simulink model "turbine_decoupled"  (R2025b)
settings: Solver=FixedStepAuto  StartTime=0.0  StopTime=399  FixedStep=Ts_inner  RelTol=1e-3
InitFcn:
  | turbine_model_constants;
values from neighbouring files (symbols this model uses):
  A = Simulink.Parameter(R.Value^2*pi)    [turbine_model_constants.m]
  beta_opt_vector = Simulink.Parameter(beta_array)    [turbine_model_constants.m]
  beta_vector = Simulink.Parameter(tables{4})    [turbine_model_constants.m]
  c_beta_dot = Simulink.Parameter(0.5)    [turbine_model_constants.m]
  c_gamma_dot = Simulink.Parameter(0.5/180*pi)    [turbine_model_constants.m]
  cp_max = Simulink.Parameter(max(cp_table.Value(:))*0.99)    [turbine_model_constants.m]
  cp_opt_keys = Simulink.Parameter(cell2mat(cp_vector))    [turbine_model_constants.m]
  cp_table = Simulink.Parameter(tables{1})    [turbine_model_constants.m]
  ct_table = Simulink.Parameter(tables{2})    [turbine_model_constants.m]
  JT = Simulink.Parameter(2.052*10^8*3)    [turbine_model_constants.m]
  lambda_opt_vector = Simulink.Parameter(lambda_array)    [turbine_model_constants.m]
  lambda_vector = Simulink.Parameter(tables{5})    [turbine_model_constants.m]
  mu = Simulink.Parameter(0.95)    [turbine_model_constants.m]
  R = Simulink.Parameter(142)    [turbine_model_constants.m]
  rho = Simulink.Parameter(1.225)    [turbine_model_constants.m]
  Ts = 1    [turbine_model_constants.m]
  Ts_inner = Simulink.Parameter(0.1)    [turbine_model_constants.m]
undefined symbols (not defined in the file or in its folder): DiscIntNeverNeededParam, f
libraries: instrumentlib x2, slpidlib x1
settings Model: Creator=kohlh  LastModifiedBy=kohlh

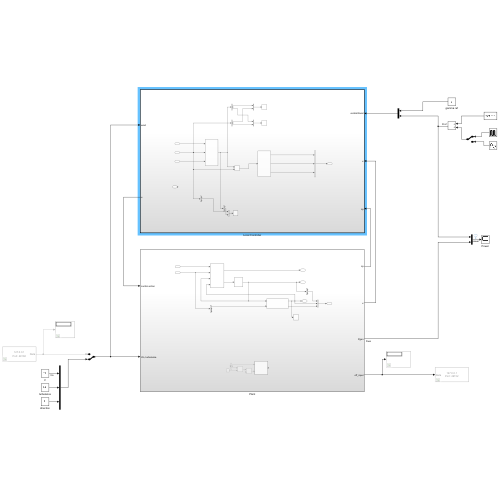
[thumbnail: Simulink's stored preview of the top-level diagram]
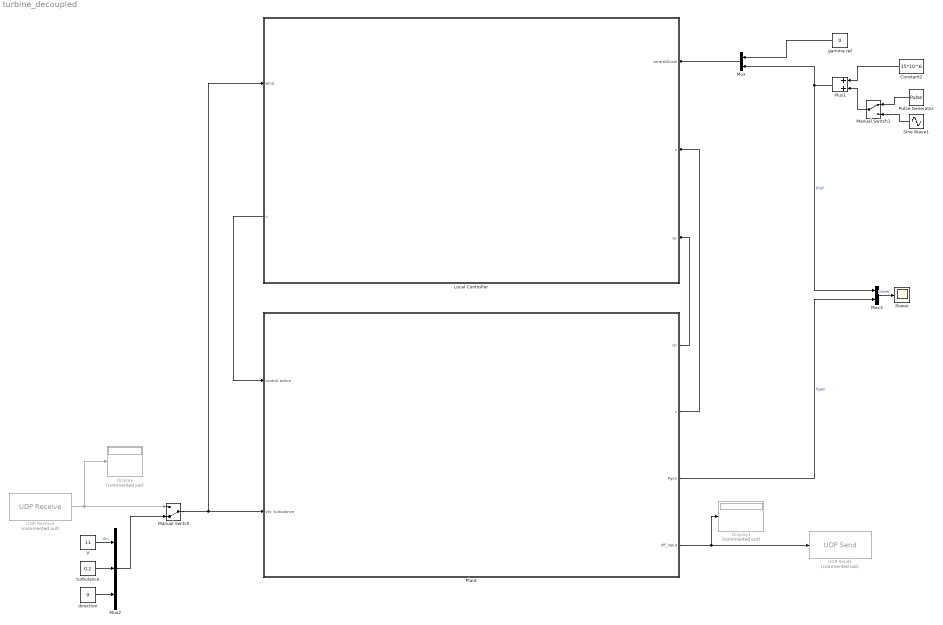
== system turbine_decoupled ==
  Constant2 : Constant  Value=15*10^6
  Display : Display  Commented=on
  Display1 : Display  Commented=on
  Local Controller : Subsystem  TreatAsAtomicUnit=on
      settings: PortSchema="{\"entries\":[{\"content\":{\"sides\":[{\"content\":{\"connectorIds\":[\"In1\",\"In2\",\"In3\"]},\"type\":\"ConnectorPlacement.EquallySpacedRectSide\",\"uuid\":\"1274bf49-ceae-40b5-8168-864c275c8277\"},{\"content\":{\"connectorIds\":[\"In4\",\"Out1\"],\"side\":\"RIGHT\"},\"type\":\"ConnectorPlacement.EquallySpacedRectSide\",\"uuid\":\"983d855e-2fb7-4029-8a1e-74d0395d6e6b\"},{\"content\":{\"side\":\"TOP\"},\"type\":\"ConnectorPlacement.EquallySpacedRectSide\",\"uuid\":\"78e40a3c-46aa-4158-bc61-97e5b88f823b\"},{\"content\":{\"side\":\"BOTTOM\"},\"type\":\"ConnectorPlacement.EquallySpacedRectSide\",\"uuid\":\"db79cd87-5583-4254-9385-067380eca232\"}]},\"type\":\"ConnectorPlacement.EquallySpacedConnector\",\"uuid\":\"902a270f-1fdc-458f-b9eb-4015978e6616\"}],\"packageUris\":[\"http://schema.mathworks.com/mf0/Connector/R2020b\"],\"version\":\"1.0\"}"
  Manual Switch : ManualSwitch  CurrentSetting=0
  Manual Switch1 : ManualSwitch
  Mux : Mux  Inputs=2
  Mux2 : Mux  Inputs=3
  Mux3 : Mux  Inputs=2
  Plant : Subsystem
  Plus1 : Sum
  Power : Scope
      settings: ActiveDisplayYMinimum=-8.3745470708276331E+6  ActiveDisplayYMaximum=3.1326975350164406E+7  DataLoggingVariableName=ScopeData4
  Pulse Generator : DiscretePulseGenerator  PulseType=Time based  Amplitude=5*10^6  Period=400  PulseWidth=50
  Sine Wave1 : Sin  Amplitude=5*10^6  Frequency=3.24/1000  SampleTime=0
  UDP Receive : instrumentlib/UDP Receive  Commented=on  LocalAddress=127.0.0.1  LocalPort=49160  EnablePortSharing=off  Host=127.0.0.1  Port=49152  GetLatestData=off  DataSize=3  DataType=double  ASCIIFormatting=%f,  Terminator=LF  CustomTerminator=10  ByteOrder=big-endian  EnableBlockingMode=on  Timeout=10  SampleTime=Ts  SimulateUsing=Interpreted execution
  UDP Send1 : instrumentlib/UDP Send  Commented=on  Host=127.0.0.1  Port=49152  LocalAddress=0.0.0.0  LocalPort=-1  EnablePortSharing=off  OutputDatagramPacketSize=512  ByteOrder=big-endian  EnableBlockingMode=on  SimulateUsing=Interpreted execution
  V : Constant  Value=11
  direction : Constant  Value=0
  gamma ref : Constant  Value=0
  turbulance : Constant  Value=0.2
  wires:
  Plant/2(x) -> Local Controller/2(x)
  Local Controller/1(u) -> Plant/1(control action)
  Plant/3(Pgen) -> Mux3/2  "Pgen"
  Manual Switch/1 -> Local Controller/4(wind), Plant/2("Vin, turbulance")
  Manual Switch1/1 -> Plus1/2
  Sine Wave1/1 -> Manual Switch1/2
  Constant2/1 -> Plus1/1
  V/1 -> Mux2/1  "Vin"
  turbulance/1 -> Mux2/2
  Mux3/1 -> Power/1  "power"
  Plant/1(cp) -> Local Controller/3(cp)
  Pulse Generator/1 -> Manual Switch1/1
  direction/1 -> Mux2/3
  Mux2/1 -> Manual Switch/2
  Plus1/1 -> Mux/2, Mux3/1  "Pref"
  gamma ref/1 -> Mux/1
  Mux/1 -> Local Controller/1(central2local)
  Plant/4(off_input) -> Display1/1, UDP Send1/1
  UDP Receive/1 -> Manual Switch/1, Display/1

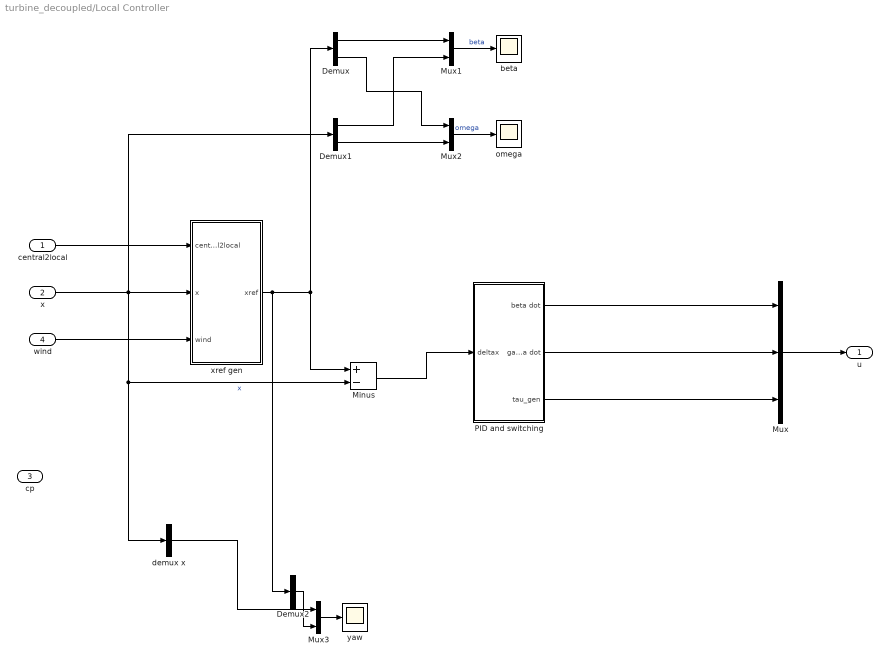
== system turbine_decoupled/Local Controller ==
  central2local : Inport
  x : Inport  Port=2
  cp : Inport  Port=3
  wind : Inport  Port=4
  Demux : Demux  Outputs=3
  Demux1 : Demux  Outputs=3
  Demux2 : Demux  Outputs=3
  Minus : Sum  Inputs=+-
  Mux : Mux  Inputs=3
  Mux1 : Mux  Inputs=2
  Mux2 : Mux  Inputs=2
  Mux3 : Mux  Inputs=2
  PID and switching : Subsystem
  beta : Scope
      settings: ActiveDisplayYMinimum=-0.675  ActiveDisplayYMaximum=6.0750000000000011
  demux x : Demux  Outputs=3
  omega : Scope
      settings: ActiveDisplayYMinimum=-0.34183960096413279  ActiveDisplayYMaximum=3.0765564086771957
  xref gen : MATLAB Function  TreatAsAtomicUnit=on
  yaw : Scope
      settings: ActiveDisplayYMinimum=-5.7595100216969257  ActiveDisplayYMaximum=9.1647979110356328  DataLoggingVariableName=ScopeData3
  u : Outport
  wires:
  central2local/1 -> xref gen/1(central2local)
  xref gen/1(xref) -> Demux2/1, Minus/1, Demux/1
  Mux/1 -> u/1
  PID and switching/1(beta dot) -> Mux/1
  PID and switching/2(gamma dot) -> Mux/2
  x/1 -> demux x/1, Minus/2, Demux1/1, xref gen/2(x)  "x"
  wind/1 -> xref gen/3(wind)
  Mux1/1 -> beta/1  "beta"
  Mux2/1 -> omega/1  "omega"
  Demux/1 -> Mux1/1
  Demux1/3 -> Mux2/2
  Demux1/1 -> Mux1/2
  Demux/3 -> Mux2/1
  demux x/2 -> Mux3/1
  Mux3/1 -> yaw/1
  Demux2/2 -> Mux3/2
  Minus/1 -> PID and switching/1(deltax)
  PID and switching/3(tau_gen) -> Mux/3

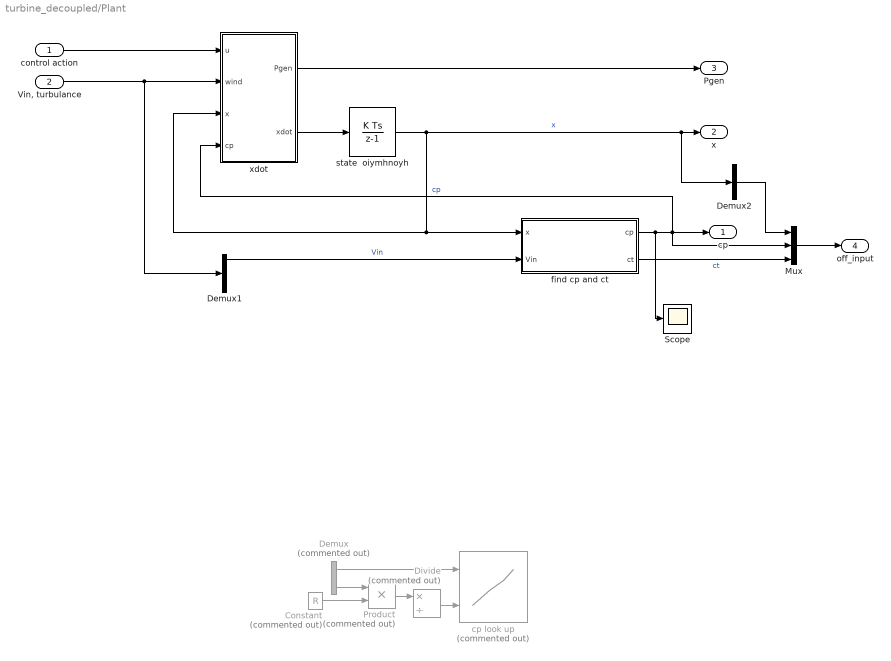
== system turbine_decoupled/Plant ==
  control action : Inport
  "Vin, turbulance" : Inport  Port=2
  Constant : Constant  Commented=on  Value=R
  Demux : Demux  Commented=on  Outputs=3
  Demux1 : Demux  Outputs=3
  Demux2 : Demux  Outputs=3
  Divide : Product  Commented=on  Inputs=*/
  Mux : Mux  Inputs=3
  Product : Product  Commented=on
  Scope : Scope
      settings: ActiveDisplayYMinimum=-0.044951731714988244  ActiveDisplayYMaximum=0.53080020994082311  DataLoggingVariableName=ScopeData2
  cp look up : Lookup_n-D  Commented=on  BreakpointsForDimension1="[2.0    2.632    3.263    3.895    4.526    5.158    5.789    6.421    7.053    7.684    8.316    8.947    9.579    10.21    10.84    11.47    12.11    12.74    13.37    14.0]"  BreakpointsForDimension2="[-5.0   -2.368   0.2632   2.895   5.526   8.158   10.79   13.42   16.05   18.68   21.32   23.95   26.58   29.21   31.84   34.47   37.11   39.74   42.37   45.0]"  Table=|  ExtrapMethod=Clip  UseLastTableValue=on  InternalRulePriority=Speed  RndMeth=Simplest
      | [0.004183   0.008552   0.013076   0.017954   0.023246   0.028797   0.034398   0.040294   0.047129   0.053808   0.057993   0.058951   0.056907   0.052360   0.045879   0.038003   0.029036   0.019157   0.008446   -0.002755;   
      | 0.014528   0.023851   0.033841   0.044146   0.054123   0.065155   0.078342   0.088804   0.092608   0.090398   0.083572   0.073569   0.061407   0.047713   0.032764   0.016578   -0.000877   -0.018725   -0.033888   -0.044500   ;
      | 0.035083   0.052168   0.068563   0.085329   0.106367   0.126719   0.134796   0.131887   0.121585   0.106602   0.088719   0.068791   0.047244   0.024090   -0.000932   -0.027634   -0.052318   -0.069329   -0.080611   -0.089918   ;
      | 0.067497   0.092129   0.118436   0.152867   0.179485   0.184226   0.174698   0.156824   0.134064   0.108187   0.079927   0.049652   0.017175   -0.018082   -0.055707   -0.088857   -0.109352   -0.123217   -0.135333   -0.145575   ;
      | 0.109296   0.146828   0.196926   0.234101   0.238344   0.224125   0.199908   0.169919   0.136059   0.099086   0.059484   0.016949   -0.029396   -0.079729   -0.125829   -0.154070   -0.171841   -0.188440   -0.202090   -0.218450   ;
      | 0.163377   0.228953   0.285997   0.296203   0.280800   0.252396   0.216375   0.175204   0.129721   0.080591   0.027761   -0.029928   -0.093612   -0.157541   -0.201469   -0.225214   -0.247672   -0.266413   -0.286681   -0.311430   ;
      | 0.239912   0.324864   0.352474   0.342011   0.313180   0.273733   0.226976   0.174102   0.115954   0.053053   -0.015678   -0.091943   -0.174928   -0.244852   -0.282403   -0.310236   -0.337440   -0.361077   -0.393459   -0.426107   ;
      | 0.333600   0.395237   0.400481   0.377508   0.339368   0.290473   0.232755   0.167308   0.095180   0.016217   -0.071529   -0.170062   -0.270275   -0.338551   -0.374587   -0.411011   -0.442593   -0.477339   -0.524911   -0.565339   ;
      | 0.402440   0.440975   0.435173   0.406148   0.361342   0.303497   0.234290   0.155195   0.067363   -0.030370   -0.140598   -0.264045   -0.376585   -0.440727   -0.482770   -0.527917   -0.566739   -0.618765   -0.682470   -0.732169   ;
      | 0.432644   0.465056   0.459322   0.429497   0.379883   0.313246   0.231892   0.137909   0.032249   -0.087249   -0.223737   -0.372811   -0.492396   -0.554948   -0.608268   -0.662234   -0.713574   -0.787600   -0.867515   -0.929642   ;
      | 0.422710   0.465336   0.473606   0.448041   0.395244   0.319950   0.225727   0.115425   -0.010492   -0.155017   -0.321542   -0.495464   -0.618709   -0.684596   -0.751969   -0.816482   -0.886063   -0.985630   -1.082210   -1.161646   ;
      | 0.396284   0.443496   0.476394   0.461471   0.407453   0.323743   0.215870   0.087597   -0.061232   -0.234314   -0.434191   -0.631316   -0.757268   -0.831922   -0.915179   -0.993282   -1.086290   -1.214677   -1.328998   -1.433710   ;
      | 0.364006   0.418141   0.464679   0.468984   0.416461   0.324694   0.202328   0.054221   -0.120379   -0.325817   -0.561780   -0.780269   -0.909948   -0.998339   -1.099511   -1.194694   -1.316095   -1.476528   -1.610379   -1.752233   ;
      | 0.325277   0.390074   0.445602   0.469191   0.422138   0.322825   0.185054   0.015070   -0.188371   -0.430168   -0.704475   -0.942914   -1.078621   -1.185143   -1.306571   -1.422529   -1.577451   -1.773037   -1.929044   -2.123730   ;
      | 0.279585   0.358093   0.423416   0.460215   0.424264   0.318123   0.163968   -0.030112   -0.265678   -0.547899   -0.862513   -1.120134   -1.265031   -1.393761   -1.537797   -1.678629   -1.872403   -2.106073   -2.288499   -2.553238   ;
      | 0.226506   0.321424   0.398243   0.444906   0.422523   0.310551   0.138956   -0.081606   -0.352786   -0.679510   -1.036172   -1.312951   -1.470710   -1.625580   -1.794579   -1.964822   -2.202969   -2.477562   -2.692792   -3.044259   ;
      | 0.165936   0.279533   0.369843   0.426424   0.416456   0.300051   0.109877   -0.139708   -0.450192   -0.825504   -1.225802   -1.522456   -1.697101   -1.881847   -2.078375   -2.282902   -2.571085   -2.889486   -3.146140   -3.599615   ;
      | 0.099525   0.232060   0.337924   0.405286   0.405362   0.286537   0.076570   -0.204724   -0.558401   -0.986390   -1.431931   -1.749759   -1.945607   -2.163742   -2.390678   -2.634632   -2.978667   -3.343918   -3.652816   -4.221737   ;
      | 0.037721   0.178916   0.302216   0.381569   0.388958   0.269906   0.038866   -0.276967   -0.677907   -1.162688   -1.655209   -1.995993   -2.217511   -2.472435   -2.732975   -3.021755   -3.427648   -3.842988   -4.217100   -4.912785   ;
      | -0.007435   0.121264   0.262494   0.355204   0.368798   0.250044   -0.003414   -0.356756   -0.809181   -1.354921   -1.896339   -2.262341   -2.513981   -2.809119   -3.106746   -3.446005   -3.919962   -4.388970   -4.843093   -5.674879]
      settings: InputPortMap=u0,u1
  find cp and ct : MATLAB Function  TreatAsAtomicUnit=on
  state  oiymhnoyh : DiscreteIntegrator  InitialCondition=[0,0,0]  SampleTime=-1  ICPrevOutput=DiscIntNeverNeededParam  ICPrevScaledInput=DiscIntNeverNeededParam
  xdot : MATLAB Function  TreatAsAtomicUnit=on
  cp : Outport
  x : Outport  Port=2
  Pgen : Outport  Port=3
  off_input : Outport  Port=4
  wires:
  "Vin, turbulance"/1 -> xdot/2(wind), Demux1/1
  xdot/2(xdot) -> state  oiymhnoyh/1
  state  oiymhnoyh/1 -> Demux2/1, x/1, find cp and ct/1(x), xdot/3(x)  "x"
  control action/1 -> xdot/1(u)
  Demux/1 -> cp look up/1
  Demux/3 -> Product/1
  Constant/1 -> Product/2
  Product/1 -> Divide/1
  Divide/1 -> cp look up/2
  xdot/1(Pgen) -> Pgen/1
  Demux1/1 -> find cp and ct/2(Vin)  "Vin"
  find cp and ct/1(cp) -> Scope/1, Mux/2, cp/1, xdot/4(cp)  "cp"
  find cp and ct/2(ct) -> Mux/3  "ct"
  Demux2/2 -> Mux/1
  Mux/1 -> off_input/1

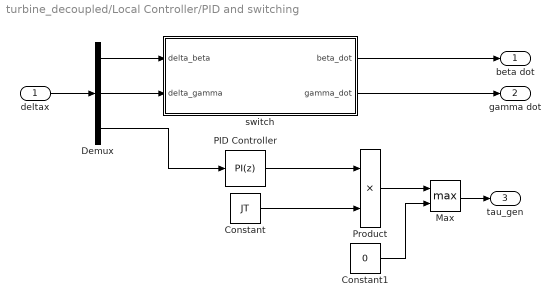
== system turbine_decoupled/Local Controller/PID and switching ==
  deltax : Inport
  Constant : Constant  Value=JT
  Constant1 : Constant  Value=0
  Demux : Demux  Outputs=3
  Max : MinMax  Function=max  Inputs=2
  PID Controller : slpidlib/PID Controller  Controller=PI  Form=Parallel  TimeDomain=Discrete-time  UseExternalTs=off  SampleTime=-1  IntegratorMethod=Forward Euler  FilterMethod=Forward Euler  ControllerParametersSource=internal  P=-0.01  I=-0.001  UseKiTs=off  D=0  UseExternalDerivativeSource=off  N=100  UseFilter=on  TunerSelectOption=Transfer Function Based (PID Tuner App)  InitialConditionSource=internal  InitialConditionForIntegrator=0  InitialConditionForFilter=0  DifferentiatorICPrevScaledInput=0  ExternalReset=none  TrackingMode=off  Kt=1  LimitOutput=off  SatLimitsSource=internal  UpperSaturationLimit=inf  LowerSaturationLimit=-inf  LinearizeAsGain=on  AntiWindupMode=none  Kb=1  LimitIntegrator=off  UpperIntegratorSaturationLimit=inf  LowerIntegratorSaturationLimit=-inf  POutMin=[]  POutMax=[]  IOutMin=[]  IOutMax=[]  DOutMin=[]  DOutMax=[]  NOutMin=[]  NOutMax=[]  SumOutMin=[]  SumOutMax=[]  SaturationOutMin=[]  SaturationOutMax=[]  PParamMin=[]  PParamMax=[]  IParamMin=[]  IParamMax=[]  DParamMin=[]  DParamMax=[]  NParamMin=[]  NParamMax=[]  KbParamMin=[]  KbParamMax=[]  KtParamMin=[]  KtParamMax=[]  KbOutMin=[]  KbOutMax=[]  KtOutMin=[]  KtOutMax=[]  IntegratorOutMin=[]  IntegratorOutMax=[]  FilterOutMin=[]  FilterOutMax=[]  SumI1OutMin=[]  SumI1OutMax=[]  SumI2OutMin=[]  SumI2OutMax=[]  SumI3OutMin=[]  SumI3OutMax=[]  SumI4OutMin=[]  SumI4OutMax=[]  SumDOutMin=[]  SumDOutMax=[]  DifferentiatorOutMin=[]  DifferentiatorOutMax=[]  FilterDiffOutCoefMin=[]  FilterDiffOutCoefMax=[]  ReciprocalOutMin=[]  ReciprocalOutMax=[]  SumDenOutMin=[]  SumDenOutMax=[]  SumNumOutMin=[]  SumNumOutMax=[]  DivideOutMin=[]  DivideOutMax=[]  UdiffTsProdOutMin=[]  UdiffTsProdOutMax=[]  NTsProdOutMin=[]  NTsProdOutMax=[]  UintegralTsProdOutMin=[]  UintegralTsProdOutMax=[]  UngainTsProdOutMin=[]  UngainTsProdOutMax=[]  ClampingZeroOutDataTypeStr=Inherit: Inherit via back propagation  ClampingZeroOutMin=[]  ClampingZeroOutMax=[]  FilterDenConstantOutDataTypeStr=Inherit: Inherit via back propagation  FilterDenConstantOutMin=[]  FilterDenConstantOutMax=[]  PCopyOutDataTypeStr=Inherit: Inherit via back propagation  PCopyOutMin=[]  PCopyOutMax=[]  NCopyOutDataTypeStr=Inherit: Inherit via back propagation  NCopyOutMin=[]  NCopyOutMax=[]  IntegratorContinuousStateAttributes=''  IntegratorStateMustResolveToSignalObject=off  IntegratorRTWStateStorageClass=Auto  FilterContinuousStateAttributes=''  FilterStateMustResolveToSignalObject=off  FilterRTWStateStorageClass=Auto  ParallelPVariant=InternalParameters  IdealPVariant=Disabled  IVariant=InternalParameters  DVariant=Disabled  IntegratorVariant=Discrete  SatVariant=Disabled  AWVariant=Passthrough  PCopyVariant=Disabled  TRVariant=Disabled  FdbkBlocksVariant=Forward  IdealPFdbkVariant=Disabled  SatFdbkVariant=Disabled  DerivativeFilterVariant=Disabled  NVariant=Disabled  NCopyVariant=Disabled_SignalSpec  FilterICVariant=Disabled  IntegratorICVariant=InternalICs  ExternalResetVariant=Disabled  TRSumVariant=Passthrough  SumFdbkVariant=Disabled  SumVariant=Sum_PI  TsampFilterVariant=InternalTs  TsampNgainVariant=Passthrough  TsampIntegralVariant=Disabled_SignalSpec  ExternalSaturationOutDataTypeStr=Inherit: Same as second input  DerivativeSourceVariant=Disabled  PreIntVariant=InternalPreInt
  Product : Product
  switch : MATLAB Function  TreatAsAtomicUnit=on
  beta dot : Outport
  gamma dot : Outport  Port=2
  tau_gen : Outport  Port=3
  wires:
  deltax/1 -> Demux/1
  Demux/1 -> switch/1(delta_beta)
  Demux/2 -> switch/2(delta_gamma)
  switch/2(gamma_dot) -> gamma dot/1
  switch/1(beta_dot) -> beta dot/1
  Demux/3 -> PID Controller/1
  PID Controller/1 -> Product/1
  Constant/1 -> Product/2
  Product/1 -> Max/1
  Constant1/1 -> Max/2
  Max/1 -> tau_gen/1

== matlab function turbine_decoupled/Local Controller/PID and switching/switch ==
  data: beta_dot output; delta_beta input; gamma_dot output; delta_gamma input; c_beta_dot parameter; c_gamma_dot parameter; Ts_inner parameter
function [beta_dot, gamma_dot]= switch_controller(delta_beta, delta_gamma, c_beta_dot, c_gamma_dot, Ts_inner)


if abs(delta_beta) > 0.5*Ts_inner*c_beta_dot
    if delta_beta > 0
        beta_dot = c_beta_dot;
    else
        beta_dot = -c_beta_dot;
    end
else
    beta_dot = 0;
end

if abs(delta_gamma) > 0.5*Ts_inner*c_gamma_dot
    if delta_gamma > 0
        gamma_dot = c_gamma_dot;
    else
        gamma_dot = -c_gamma_dot;
    end
else
    gamma_dot = 0;
end

end

== matlab function turbine_decoupled/Plant/xdot ==
  data: Pgen output; u input; xdot output; wind input; x input; cp input; JT parameter; A parameter; rho parameter; mu parameter
function [Pgen, xdot] = fcn(u, wind, x, cp, JT, A, rho, mu)

Vin = wind(1);
turbulance = 1-wind(2);
wind_direction = wind(3);

beta_dot = u(1);
gamma_dot = u(2);
tau_gen = u(3);

gamma = x(2);
omega = x(3);

%eliminating division by 0
if omega < 0.1 && omega >= 0
    omega = 0.1;
    tau_gen = 0;
    % if there is no motion backwards acc due to tau aero is not allowed
    tau_aero = max(0, cp * Vin^3 * rho * A * 1/2 * turbulance * cos(wind_direction-gamma)^3 / omega);
elseif omega < 0
    tau_aero = abs(cp * Vin^3 * rho * A * 1/2 * turbulance * cos(wind_direction-gamma)^3 / omega);
    tau_gen = 0;
else
    tau_aero = cp * Vin^3 * rho * A * 1/2 * turbulance * cos(wind_direction-gamma)^3 / omega;
end

omega_dot = (tau_aero - tau_gen)/JT;

xdot = [beta_dot, gamma_dot, omega_dot];
Pgen = tau_gen * omega * mu;

end

== matlab function turbine_decoupled/Local Controller/xref gen ==
  data: central2local input; x input; wind input; xref output; mu parameter; lambda_vector parameter; beta_vector parameter; cp_table parameter; R parameter; rho parameter; A parameter; cp_max parameter; cp_opt_keys parameter; beta_opt_vector parameter; c_beta_dot parameter; Ts_inner parameter; lambda_opt_vector parameter
function xref  = xrefgen(central2local,  x, wind, mu, lambda_vector, beta_vector, cp_table, R, rho, A, cp_max, cp_opt_keys, beta_opt_vector, c_beta_dot, Ts_inner, lambda_opt_vector)
    Vin = wind(1);
    turbulance = 1-wind(2);
    wind_direction = wind(3);

    Pref = central2local(2);
    gamma_ref = wind_direction; %central2local(1);
    
    beta = x(1);
    gamma = x(2);
    omega = x(3);
    
    %cap cpref to avoid oscillation at the boundary
    Pref = max(min(Pref, (1/2 * Vin^3 * rho * A * mu * turbulance*cos(wind_direction - gamma)^3)*cp_max),0);
    if cos(wind_direction - gamma) > 0
        cpref = Pref/(1/2 * Vin^3 * rho * A * mu * turbulance*cos(wind_direction - gamma)^3);
    else
        cpref = 0;
    end

    
    %find closest cp opt key that is larger than cpref
    [closest_cp, ~] = min(abs((cp_opt_keys >= cpref) - cpref));
    [~,closest_cp_index] = min(abs(cp_opt_keys - closest_cp));
    beta_opt = beta_opt_vector(closest_cp_index);
    %find beta that is achieveable with delta beta
    deltabeta = c_beta_dot * Ts_inner;
    beta_over = ceil((beta_opt - beta)/deltabeta) * deltabeta + beta;
    beta_under = floor((beta_opt - beta)/deltabeta) * deltabeta + beta;

    beta_ref = beta_under;

    cp_at_beta_opt = NaN;
    for i = 1:length(beta_vector)-1
        if beta_vector(i) <= beta_ref && beta_vector(i+1) >= beta_ref
            cp_at_beta_opt = cp_table(1:end,i) * abs((beta_ref - beta_vector(i+1))/(beta_vector(i+1) - beta_vector(i))) + cp_table(1:end,i+1) * abs((beta_ref - beta_vector(i))/(beta_vector(i+1) - beta_vector(i)));
            break
        end
    end

    lambda_ref = NaN;
    for i = 1:length(beta_vector)-1
        if (cp_at_beta_opt(i) <= cpref && cp_at_beta_opt(i+1) >= cpref) || (cp_at_beta_opt(i+1) <= cpref && cp_at_beta_opt(i) >= cpref)
            lambda_ref = lambda_vector(i) * abs((cpref - cp_at_beta_opt(i+1))/(cp_at_beta_opt(i+1) - cp_at_beta_opt(i))) + lambda_vector(i+1) * abs((cpref - cp_at_beta_opt(i))/(cp_at_beta_opt(i+1) - cp_at_beta_opt(i)));
            break
        end
    end

    if isnan(lambda_ref)
        beta_ref = beta_over;

        for i = 1:length(beta_vector)-1
            if beta_vector(i) <= beta_ref && beta_vector(i+1) >= beta_ref
                cp_at_beta_opt = cp_table(1:end,i) * abs((beta_ref - beta_vector(i+1))/(beta_vector(i+1) - beta_vector(i))) + cp_table(1:end,i+1) * abs((beta_ref - beta_vector(i))/(beta_vector(i+1) - beta_vector(i)));
                break
            end
        end

        for i = 1:length(beta_vector)-1
            if (cp_at_beta_opt(i) <= cpref && cp_at_beta_opt(i+1) >= cpref) || (cp_at_beta_opt(i+1) <= cpref && cp_at_beta_opt(i) >= cpref)
                lambda_ref = lambda_vector(i) * abs((cpref - cp_at_beta_opt(i+1))/(cp_at_beta_opt(i+1) - cp_at_beta_opt(i))) + lambda_vector(i+1) * abs((cpref - cp_at_beta_opt(i))/(cp_at_beta_opt(i+1) - cp_at_beta_opt(i)));
                break
            end
        end
    end
    if isnan(lambda_ref)
        beta_ref = beta_opt;
        for i = 1:length(beta_vector)-1
            if beta_vector(i) <= beta_ref && beta_vector(i+1) >= beta_ref
                cp_at_beta_opt = cp_table(1:end,i) * abs((beta_ref - beta_vector(i+1))/(beta_vector(i+1) - beta_vector(i))) + cp_table(1:end,i+1) * abs((beta_ref - beta_vector(i))/(beta_vector(i+1) - beta_vector(i)));
                break
            end
        end

        for i = 1:length(beta_vector)-1
            if (cp_at_beta_opt(i) <= cpref && cp_at_beta_opt(i+1) >= cpref) || (cp_at_beta_opt(i+1) <= cpref && cp_at_beta_opt(i) >= cpref)
                lambda_ref = lambda_vector(i) * abs((cpref - cp_at_beta_opt(i+1))/(cp_at_beta_opt(i+1) - cp_at_beta_opt(i))) + lambda_vector(i+1) * abs((cpref - cp_at_beta_opt(i))/(cp_at_beta_opt(i+1) - cp_at_beta_opt(i)));
                break
            end
        end
    end
    if isnan(lambda_ref)
        lambda_ref = lambda_opt_vector(closest_cp_index);
    end
    
    omega_ref = lambda_ref * Vin / R;   
    xref = [beta_ref, gamma_ref, omega_ref];
end

== matlab function turbine_decoupled/Plant/find cp and ct ==
  data: x input; cp output; ct output; Vin input; R parameter; beta_vector parameter; lambda_vector parameter; cp_table parameter; ct_table parameter
function [cp, ct] = lookup(x, Vin, R, beta_vector, lambda_vector, cp_table, ct_table)
beta = x(1);
omega = x(3);
lambda = omega * R/ Vin;

beta_index_under = 0;
for i=1:length(beta_vector)-1
    if beta>beta_vector(i)
        beta_index_under = i;
    end
end

lambda_index_under = 0;
for i=1:length(lambda_vector)-1
    if lambda>lambda_vector(i)
        lambda_index_under = i;
    end
end

if beta_index_under == 0
    beta_under_coef = 1;
    beta_index_under = 1;
elseif beta > beta_vector(end)
    beta_under_coef = 0;
else
    beta_under_coef = abs((beta_vector(beta_index_under+1) - beta)/(beta_vector(beta_index_under) - beta_vector(beta_index_under+1)));
end

if lambda_index_under == 0
    lambda_under_coef = 1;
    lambda_index_under = 1;
elseif lambda > lambda_vector(end)
    lambda_under_coef = 0;
else
    lambda_under_coef = abs((lambda_vector(lambda_index_under+1) - lambda)/(lambda_vector(lambda_index_under) - lambda_vector(lambda_index_under+1)));
end

cp = cp_table(lambda_index_under, beta_index_under) * (beta_under_coef * lambda_under_coef) ...
    + cp_table(lambda_index_under+1, beta_index_under) * ((1 - lambda_under_coef) * beta_under_coef) ...
    + cp_table(lambda_index_under, beta_index_under+1) * (lambda_under_coef * (1 - beta_under_coef)) ...
    + cp_table(lambda_index_under+1, beta_index_under+1) * ((1 - lambda_under_coef) * (1 - beta_under_coef));

ct = ct_table(lambda_index_under, beta_index_under) * (beta_under_coef * lambda_under_coef) ...
    + ct_table(lambda_index_under+1, beta_index_under) * ((1 - lambda_under_coef) * beta_under_coef) ...
    + ct_table(lambda_index_under, beta_index_under+1) * (lambda_under_coef * (1 - beta_under_coef)) ...
    + ct_table(lambda_index_under+1, beta_index_under+1) * ((1 - lambda_under_coef) * (1 - beta_under_coef));
end
